simulink model "rectify"  (R2020b)
settings: Solver=VariableStepAuto  StartTime=0.0  StopTime=10.0  RelTol=1e-3
settings Model: Creator=Fong  LastModifiedBy=Fong

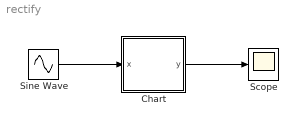
== system rectify ==
  Chart : Stateflow chart  TreatAsAtomicUnit=on
  Scope : Scope
  Sine Wave : Sin  SampleTime=0.2
  wires:
  Sine Wave/1 -> Chart/1(x)
  Chart/1(y) -> Scope/1

== stateflow chart rectify/Chart ==
  state On
    y = x;
  state Off
    y = 0;
  (default) -> On
  On -> Off : [x<t0]
  Off -> On : [x>=t0]
  data: x input double; y output single; t0 constant fixdt(1,5,2) =0
